simulink model "d_gradient_sim_sol"  (R2023b)
settings: Solver=ode3  StartTime=0.0  StopTime=200  FixedStep=0.01  RelTol=1e-3
values from neighbouring files (symbols this model uses):
  a0 = k/m    (= 0.5)    [MSD_parest_par_sol.m]    (also in d_pend_par_sol.m = 9.8)
  a1 = d/m    (= 0.01)    [MSD_parest_par_sol.m]    (also in d_pend_par_sol.m = 0.002)
  A_F = A-B*K    [MSD_parest_par_sol.m]
  b = 1/m    (= 0.1)    [MSD_parest_par_sol.m]    (also in d_pend_par_sol.m = 0.02)
  B_F = [ 0 ; 0 ; -A_F(3,1)]    [MSD_parest_par_sol.m]
  C_F0 = [ 1 0 0 ]    [MSD_parest_par_sol.m]
  C_F1 = [ 0 1 0 ]    [MSD_parest_par_sol.m]
  C_F2 = [ 0 0 1 ]    [MSD_parest_par_sol.m]
  d = 0.1    [MSD_parest_par_sol.m]    (also in d_pend_par_sol.m)
  k = 5    [MSD_parest_par_sol.m]
  m = 10    [MSD_parest_par_sol.m]    (also in d_pend_par_sol.m = 50)
settings Model: Creator=jerome  LastModifiedBy=jerome
settings ModelReferenceCC: EnableRefExpFcnMdlSchedulingChecks=on

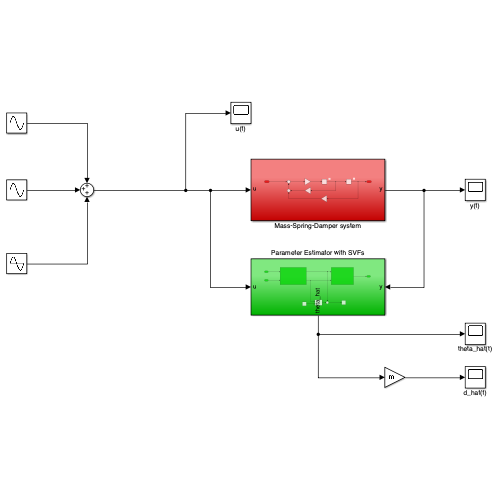
[thumbnail: Simulink's stored preview of the top-level diagram]
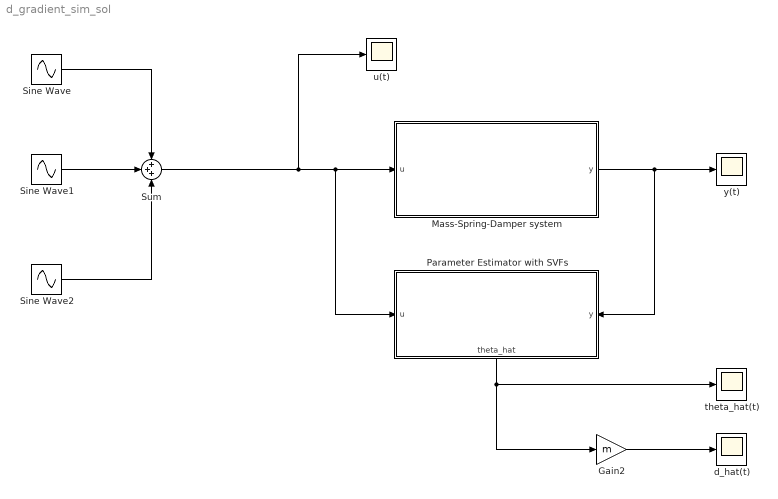
== system d_gradient_sim_sol ==
  Gain2 : Gain  Gain=m
  Mass-Spring-Damper system : Subsystem
  Parameter Estimator with SVFs : Subsystem
      settings: PortSchema="{\"entries\":[{\"content\":{\"sides\":[{\"content\":{\"connectorIds\":[\"In1\"]},\"type\":\"ConnectorPlacement.EquallySpacedRectSide\",\"uuid\":\"701dba22-d81c-4620-a4f9-4eedebec699b\"},{\"content\":{\"connectorIds\":[\"In2\"],\"side\":\"RIGHT\"},\"type\":\"ConnectorPlacement.EquallySpacedRectSide\",\"uuid\":\"14a753f7-073c-4e1b-870d-b975b59fa292\"},{\"content\":{\"connectorIds\":[],\"side\":\"TOP\"},\"type\":\"ConnectorPlacement.EquallySpacedRectSide\",\"uuid\":\"4fae71d8-e84c-4ac4-80a0-9291851fcc8b\"},{\"content\":{\"connectorIds\":[\"Out1\"],\"side\":\"BOTTOM\"},\"type\":\"ConnectorPlacement.EquallySpacedRectSide\",\"uuid\":\"a05140d0-bc49-4091-9e05-f62f82fd2c00\"}]},\"type\":\"ConnectorPlacement.EquallySpacedConnector\",\"uuid\":\"49c9441c-c785-42d3-a441-16a536410442\"}],\"packageUris\":[\"http://schema.mathworks.com/mf0/Connector/R2020b\"],\"version\":\"1.0\"}"
  Sine Wave : Sin  Phase=pi*rand  SampleTime=0
  Sine Wave1 : Sin  Frequency=2  Phase=pi/5  SampleTime=0
  Sine Wave2 : Sin  Frequency=0.5  Phase=pi/3  SampleTime=0
  Sum : Sum  Inputs=+++
  d_hat(t) : Scope
  theta_hat(t) : Scope
  u(t) : Scope
  y(t) : Scope
  wires:
  Mass-Spring-Damper system/1(y) -> Parameter Estimator with SVFs/2(y), y(t)/1
  Sum/1 -> u(t)/1, Parameter Estimator with SVFs/1(u), Mass-Spring-Damper system/1(u)
  Sine Wave/1 -> Sum/1
  Sine Wave1/1 -> Sum/2
  Sine Wave2/1 -> Sum/3
  Parameter Estimator with SVFs/1(theta_hat) -> Gain2/1, theta_hat(t)/1
  Gain2/1 -> d_hat(t)/1

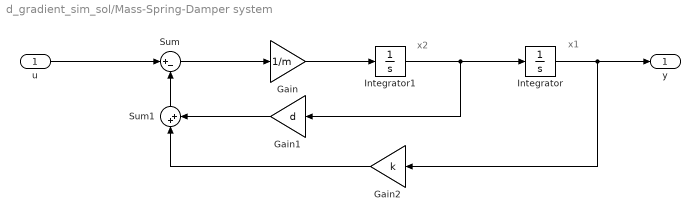
== system d_gradient_sim_sol/Mass-Spring-Damper system ==
  note: x2
  note: x1
  u : Inport
  Gain : Gain  Gain=1/m
  Gain1 : Gain  Gain=d
  Gain2 : Gain  Gain=k
  Integrator : Integrator
  Integrator1 : Integrator
  Sum : Sum  Inputs=|+-
  Sum1 : Sum  Inputs=|++
  y : Outport
  wires:
  Integrator/1 -> Gain2/1, y/1
  Integrator1/1 -> Gain1/1, Integrator/1
  u/1 -> Sum/1
  Gain/1 -> Integrator1/1
  Sum/1 -> Gain/1
  Gain1/1 -> Sum1/2
  Sum1/1 -> Sum/2
  Gain2/1 -> Sum1/1

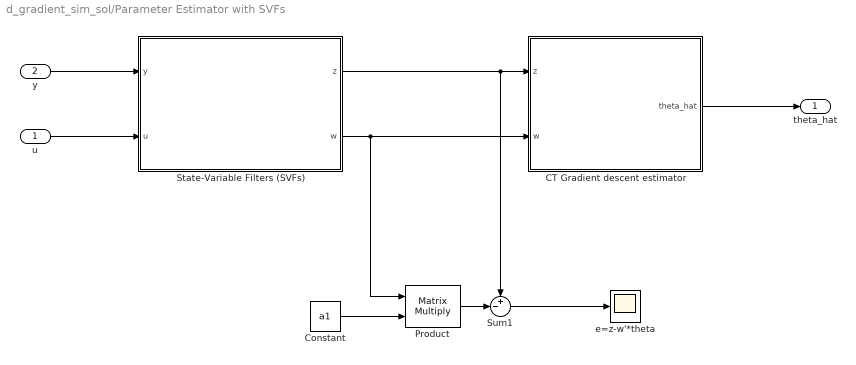
== system d_gradient_sim_sol/Parameter Estimator with SVFs ==
  u : Inport
  y : Inport  Port=2
  CT Gradient descent estimator : Subsystem
  Constant : Constant  Value=a1  VectorParams1D=off
  Product : Product  Multiplication=Matrix(*)
  State-Variable Filters (SVFs) : Subsystem
  Sum1 : Sum  Inputs=+-|
  e=z-w'*theta : Scope
  theta_hat : Outport
  wires:
  CT Gradient descent estimator/1(theta_hat) -> theta_hat/1
  State-Variable Filters (SVFs)/1(z) -> Sum1/1, CT Gradient descent estimator/1(z)
  y/1 -> State-Variable Filters (SVFs)/1(y)
  u/1 -> State-Variable Filters (SVFs)/2(u)
  Constant/1 -> Product/2
  Product/1 -> Sum1/2
  State-Variable Filters (SVFs)/2(w) -> Product/1, CT Gradient descent estimator/2(w)
  Sum1/1 -> e=z-w'*theta/1

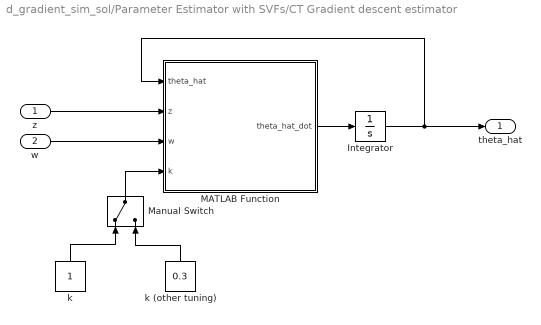
== system d_gradient_sim_sol/Parameter Estimator with SVFs/CT Gradient descent estimator ==
  z : Inport
  w : Inport  Port=2
  Integrator : Integrator
  MATLAB Function : MATLAB Function  TreatAsAtomicUnit=on
  Manual Switch : ManualSwitch
  k : Constant
  k (other tuning) : Constant  Value=0.3
  theta_hat : Outport
  wires:
  z/1 -> MATLAB Function/2(z)
  w/1 -> MATLAB Function/3(w)
  MATLAB Function/1(theta_hat_dot) -> Integrator/1
  Integrator/1 -> MATLAB Function/1(theta_hat), theta_hat/1
  Manual Switch/1 -> MATLAB Function/4(k)
  k/1 -> Manual Switch/1
  k (other tuning)/1 -> Manual Switch/2

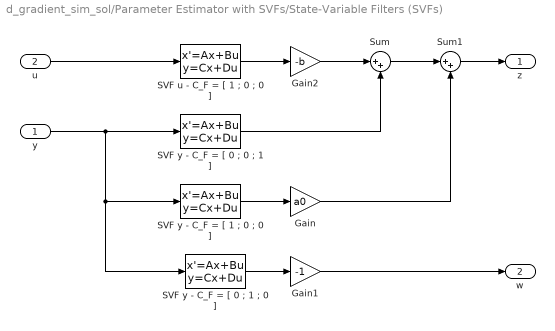
== system d_gradient_sim_sol/Parameter Estimator with SVFs/State-Variable Filters (SVFs) ==
  y : Inport
  u : Inport  Port=2
  Gain : Gain  Gain=a0
  Gain1 : Gain  Gain=-1
  Gain2 : Gain  Gain=-b
  SVF u - C_F = [ 1 ; 0 ; 0 ] : StateSpace  A=A_F  B=B_F  C=C_F0  D=0  InitialCondition=zeros(3,1)
  SVF y - C_F = [ 0 ; 0 ; 1 ] : StateSpace  A=A_F  B=B_F  C=C_F2  D=0  InitialCondition=ones(3,1)
  SVF y - C_F = [ 0 ; 1 ; 0 ] : StateSpace  A=A_F  B=B_F  C=C_F1  D=0  InitialCondition=zeros(3,1)
  SVF y - C_F = [ 1 ; 0 ; 0 ] : StateSpace  A=A_F  B=B_F  C=C_F0  D=0  InitialCondition=zeros(3,1)
  Sum : Sum  Inputs=|++
  Sum1 : Sum  Inputs=|++
  z : Outport
  w : Outport  Port=2
  wires:
  u/1 -> SVF u - C_F = [ 1 ; 0 ; 0 ]/1
  y/1 -> SVF y - C_F = [ 1 ; 0 ; 0 ]/1, SVF y - C_F = [ 0 ; 1 ; 0 ]/1, SVF y - C_F = [ 0 ; 0 ; 1 ]/1
  SVF u - C_F = [ 1 ; 0 ; 0 ]/1 -> Gain2/1
  Gain2/1 -> Sum/1
  SVF y - C_F = [ 0 ; 0 ; 1 ]/1 -> Sum/2
  Sum/1 -> Sum1/1
  Sum1/1 -> z/1
  SVF y - C_F = [ 1 ; 0 ; 0 ]/1 -> Gain/1
  Gain/1 -> Sum1/2
  Gain1/1 -> w/1
  SVF y - C_F = [ 0 ; 1 ; 0 ]/1 -> Gain1/1

== matlab function d_gradient_sim_sol/Parameter Estimator with SVFs/CT Gradient descent estimator/MATLAB Function ==
  data: theta_hat input; theta_hat_dot output; z input; w input; k input
function theta_hat_dot = fcn(theta_hat,z,w,k)

% compute Jacobian of cost function J with respect to theta_hat
dJdtheta_hat = 2*w*(w*theta_hat - z);

% basic gradient descent algorithm
theta_hat_dot = -k*dJdtheta_hat;
